simulink model "c2f_callback"  (R2019b)
settings: Solver=ode45  StartTime=0  StopTime=364  RelTol=1e-3  EnableMultiTasking=on
PreLoadFcn:
  | load bangaloreTempsC;
  | t = [0:364]';
  | bias = 32;
  | scale = 9/5;
StopFcn:
  | plot(tout, yout); grid on;
  | xlabel('Day of the year');
  | ylabel('Max temperature in ^oF');
  | title('Daily maximum temperatures in Bangalore in 2005');
settings Model: Creator=bbhattac  LastModifiedBy=khung
settings DataIOCC: ExternalInput=[t, TmaxC]  LimitDataPoints=on  LoadExternalInput=on  SaveFormat=Array  ReturnWorkspaceOutputs=off
settings OptimizationCC: ExpressionDepthLimit=2147483647  LifeSpan=inf
settings DebuggingCC: UnderspecifiedInitializationDetection=Classic  MergeDetectMultiDrivingBlocksExec=none  SolverPrmCheckMsg=warning  StateNameClashWarn=warning  SFUnexpectedBacktrackingDiag=warning  SFNoUnconditionalDefaultTransitionDiag=warning  SFExecutionAtInitializationDiag=none  ArithmeticOperatorsInVariantConditions=warning
settings HardwareCC: ProdBitPerPointer=32  ProdBitPerSizeT=32  ProdBitPerPtrDiffT=32  ProdLargestAtomicFloat=None  ProdIntDivRoundTo=Undefined  ProdEndianess=Unspecified  ProdWordSize=32  ProdHWDeviceType=32-bit Generic
settings ModelReferenceCC: PropagateSignalLabelsOutOfModel=off
settings SFSimCC: SimUseLocalCustomCode=off
settings RTWCC: RTWUseLocalCustomCode=off
settings CodeAppCC: StateflowObjectComments=on
settings GRTTargetCC: TargetLangStandard=C89/C90 (ANSI)  GeneratePreprocessorConditionals=Disable all  CombineOutputUpdateFcns=off  GRTInterface=on
settings ConfigComp: CovMetricSettings=dw  CovHtmlReporting=on  CovSaveCumulativeToWorkspaceVar=on  CovSaveSingleToWorkspaceVar=on  CovExternalEMLEnable=off

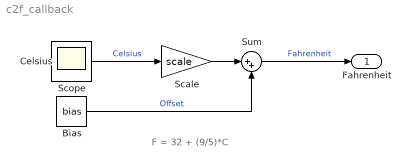
== system c2f_callback ==
  note: F = 32 + (9/5)*C
  Celsius : Inport
  Bias : Constant  Value=bias
  Scale : Gain  Gain=scale
  Sum : Sum  Inputs=|++
  Fahrenheit : Outport
  Scope : Scope
  wires:
  Scale/1 -> Sum/1
  Bias/1 -> Sum/2  "Offset"
  Sum/1 -> Fahrenheit/1  "Fahrenheit"
  Celsius/1 -> Scale/1  "Celsius"
